simulink model "q_H2"  (R2015a)
settings: Solver=ode45  StartTime=0.0  StopTime=200  RelTol=1e-3
libraries: simulink x1
settings Model: Creator=liu0563  LastModifiedBy=liu0563

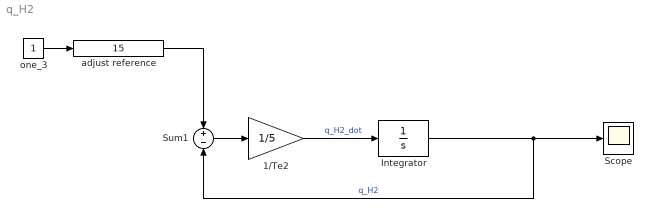
== system q_H2 ==
  1/Te2 : Gain  Gain=1/5
  Integrator : Integrator
  Scope : Scope
      settings: TimeRange=80  YMin=11.49780461031833  YMax=17.49780461031833
  Sum1 : Sum  Inputs=+-
  adjust reference : simulink/Math Operations/Slider Gain  low=1  gain=15  high=100
  one_3 : Constant
  wires:
  Integrator/1 -> Scope/1, Sum1/2  "q_H2"
  1/Te2/1 -> Integrator/1  "q_H2_dot"
  Sum1/1 -> 1/Te2/1
  adjust reference/1 -> Sum1/1
  one_3/1 -> adjust reference/1
